simulink model "SINUSOIDAL_PWM"  (R2013a)
settings: Solver=ode45  StartTime=0.0  StopTime=0.2  RelTol=1e-3
libraries: powerlib x7, simulink x3
settings Model: Creator=user  LastModifiedBy=user

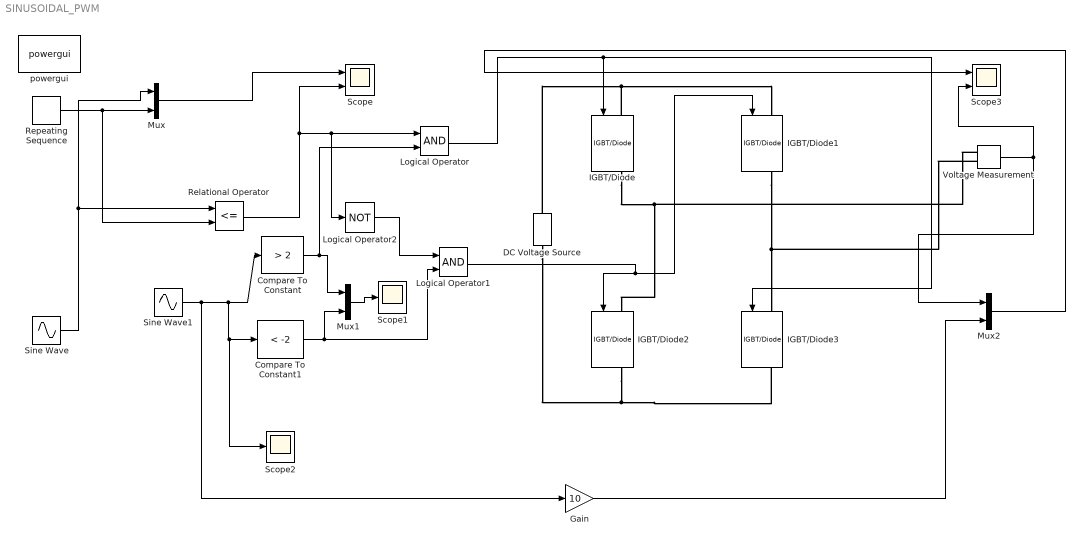
== system SINUSOIDAL_PWM ==
  Compare To Constant : simulink/Logic and Bit Operations/Compare To Constant  relop=>  const=2  OutDataTypeStr=boolean
  Compare To Constant1 : simulink/Logic and Bit Operations/Compare To Constant  relop=<  const=-2  OutDataTypeStr=boolean
  DC Voltage Source : powerlib/Electrical Sources/DC Voltage Source  Amplitude=100  Measurements=None
  Gain : Gain  Gain=10
  IGBT/Diode{,1..3} (4 alike) : powerlib/Power Electronics/IGBT//Diode  Ron=1e-3  Rs=1e5  Cs=inf  Measurements=on
  Logical Operator : Logic  AllPortsSameDT=off  OutDataTypeStr=boolean
  Logical Operator1 : Logic  AllPortsSameDT=off  OutDataTypeStr=boolean
  Logical Operator2 : Logic  Operator=NOT  AllPortsSameDT=off  OutDataTypeStr=boolean
  Mux : Mux  Inputs=2
  Mux1 : Mux  Inputs=2
  Mux2 : Mux  Inputs=2
  Relational Operator : RelationalOperator  Operator=<=  OutDataTypeStr=boolean
  Repeating Sequence : simulink/Sources/Repeating Sequence  rep_seq_t=[0 0.5e-3 1e-3]  rep_seq_y=[+10 0 -10]
  Scope : Scope  NumInputPorts=2
      settings: YMin=-5~-5  YMax=5~5
  Scope1 : Scope
  Scope2 : Scope
      settings: SaveName=ScopeData2
  Scope3 : Scope  NumInputPorts=2
      settings: YMin=-5~-5  YMax=5~5  SaveName=ScopeData3
  Sine Wave : Sin  Amplitude=10  Frequency=2*pi*50  SampleTime=1e-6
  Sine Wave1 : Sin  Amplitude=10  Frequency=2*pi*50  SampleTime=1e-6
  Voltage Measurement : powerlib/Measurements/Voltage Measurement  PhasorSimulation=off  OutputType=Complex  PSBequivalent=0
  powergui : powerlib/powergui  Priority=1  SimulationMode=Continuous  SolverType=Tustin  SampleTime=50e-6  frequency=60  SPID=off  DisableSnubberDevices=off  DisableRonSwitches=off  DisableVfSwitches=off  SwTol=0  Interpol=off  DisplayEquations=off  frequencyindice=0  Pbase=100e6  ErrMax=1e-4  Iterations=50  UnitsV=kV  UnitsW=MW  FunctionMessages=off  echomessages=off  HookPort=off  EnableUseOfTLC=off  x0status=blocks  RestoreLinks=warning  ResistiveCurrentMeasurement=off  Frange=[0:2:500]  Ylog=off  Xlog=on  ShowGrid=off  save=off  variable=ZData  ZoomFFT=off  StartTime=0.0  cycles=1  DisplayStyle=1  fundamental=60  FreqAxis=off  MaxFrequency=1000  frequencyindicesteady=1  RmsSteady=1  display=off  Ts=0  methode=off
  wires:
  Sine Wave/1 -> Mux/1, Relational Operator/1
  Repeating Sequence/1 -> Relational Operator/2, Mux/2
  Mux/1 -> Scope/1
  Relational Operator/1 -> Scope/2, Logical Operator2/1, Logical Operator/1
  Logical Operator2/1 -> Logical Operator1/1
  Compare To Constant/1 -> Logical Operator/2, Mux1/1
  Compare To Constant1/1 -> Logical Operator1/2, Mux1/2
  Mux1/1 -> Scope1/1
  Sine Wave1/1 -> Gain/1, Scope2/1, Compare To Constant1/1, Compare To Constant/1
  Logical Operator/1 -> IGBT/Diode3/1, IGBT/Diode/1
  Logical Operator1/1 -> IGBT/Diode1/1, IGBT/Diode2/1
  Gain/1 -> Mux2/2
  Voltage Measurement/1 -> Scope3/2, Mux2/1
  Mux2/1 -> Scope3/1
  connections:
  IGBT/Diode/LConn1 -- IGBT/Diode1/LConn1 -- DC Voltage Source/RConn1
  IGBT/Diode2/RConn1 -- IGBT/Diode3/RConn1 -- DC Voltage Source/LConn1
  IGBT/Diode/RConn1 -- Voltage Measurement/LConn1 -- IGBT/Diode2/LConn1
  IGBT/Diode1/RConn1 -- Voltage Measurement/LConn2 -- IGBT/Diode3/LConn1
